simulink model "lab1"  (R2017b)
settings: Solver=ode1  StartTime=0.0  StopTime=100  FixedStep=0.01  RelTol=1e-3
settings Model: Creator=mt35448  LastModifiedBy=mt35448

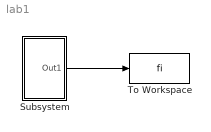
== system lab1 ==
  Subsystem : Subsystem  mask{m=10, l=3, k=1, g=10, fi0=90}
      mask prompts: m "masa"; l "dlugosc_wahadla"; k "wspl_tlumienia"; g "przyspieszenie"; fi0 "kat_wychylenia"
  To Workspace : ToWorkspace  VariableName=fi  SampleTime=-1
  wires:
  Subsystem/1(Out1) -> To Workspace/1

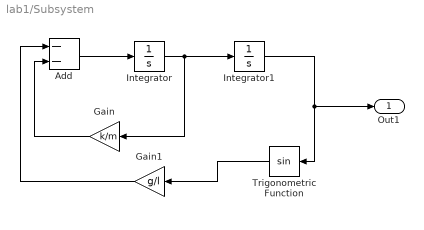
== system lab1/Subsystem ==
  Add : Sum  Inputs=--
  Gain : Gain  Gain=k/m
  Gain1 : Gain  Gain=g/l
  Integrator : Integrator
  Integrator1 : Integrator  InitialCondition=(fi0 * pi) / 180
  Trigonometric Function : Trigonometry
  Out1 : Outport
  wires:
  Integrator/1 -> Gain/1, Integrator1/1
  Add/1 -> Integrator/1
  Integrator1/1 -> Out1/1, Trigonometric Function/1
  Gain/1 -> Add/2
  Gain1/1 -> Add/1
  Trigonometric Function/1 -> Gain1/1
